simulink model "fuerza"  (R2020a)
settings: Solver=VariableStepAuto  StartTime=0.0  StopTime=2.5  RelTol=1e-3
values from neighbouring files (symbols this model uses):
  fd = 10/sqrt(2)*[1 1]    [init_control_fuerza.m]
  Ke = 1000    [init_control_fuerza.m]
  Kpf = (2*pi*freq)^2    (= 3947.84176044)    [init_control_fuerza.m]
  Kvf = 2*sqrt(Kpf)    [init_control_fuerza.m]
  Robot = Robot.perturb(0.8)    [init_control_fuerza.m]
undefined symbols (not defined in the file or in its folder): coriolis
libraries: roblocks x15, simulink x1
settings Model: Creator=Gianfranco  LastModifiedBy=Facu Molina

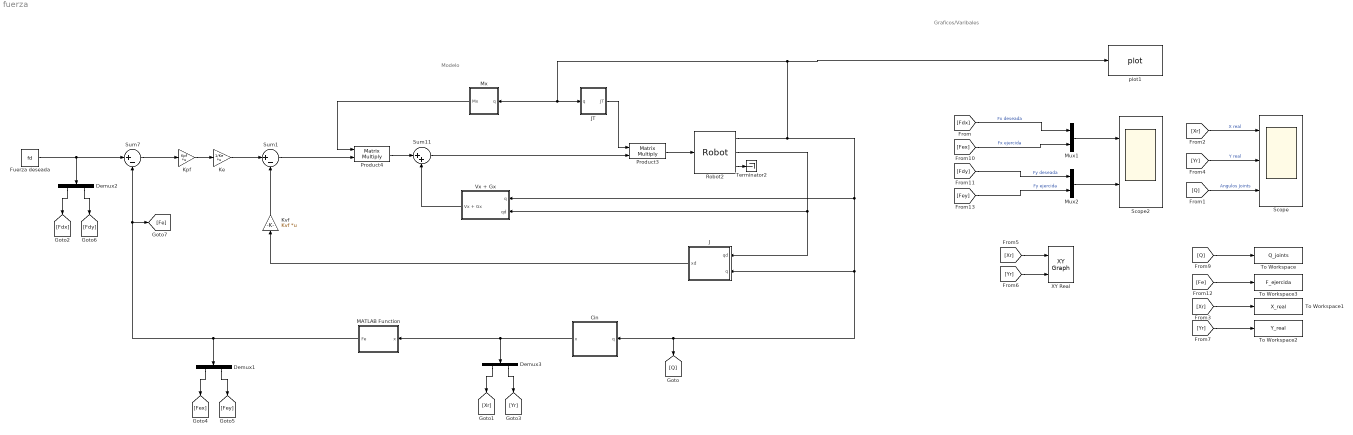
== system fuerza ==
  note: Graficos/Varibales
  note: Modelo
  Cin : Subsystem
  Demux1 : Demux  Outputs=2
  Demux2 : Demux  Outputs=2
  Demux3 : Demux  Outputs=2
  Fuerza deseada : Constant  Value=fd
  J : Subsystem
  JT : Subsystem
  Ke : Gain  Gain=1/Ke  Multiplication=Matrix(K*u)  SaturateOnIntegerOverflow=on  OutDataTypeStr=Inherit: Same as input  ParamDataTypeStr=Inherit: Same as input
  Kpf : Gain  Gain=Kpf  Multiplication=Matrix(K*u)  SaturateOnIntegerOverflow=on  OutDataTypeStr=Inherit: Same as input  ParamDataTypeStr=Inherit: Same as input
  Kvf : Gain  Gain=Kvf  Multiplication=Matrix(K*u)  SaturateOnIntegerOverflow=on  OutDataTypeStr=Inherit: Same as input  ParamDataTypeStr=Inherit: Same as input
  MATLAB Function : MATLAB Function  TreatAsAtomicUnit=on
  Mux1 : Mux  Inputs=2
  Mux2 : Mux  Inputs=2
  Mx : Subsystem
  Product3 : Product  Multiplication=Matrix(*)
  Product4 : Product  Multiplication=Matrix(*)
  Robot2 : roblocks/Arm/Robot  robot=Robot  q0=q0
      link override Integrator: InitialCondition=0
  Scope : Scope  NumInputPorts=3
  Scope2 : Scope  NumInputPorts=2
  Sum1 : Sum  Inputs=|+-  InputSameDT=on  SaturateOnIntegerOverflow=on  OutDataTypeStr=Inherit: Same as first input
  Sum11 : Sum  Inputs=|++  InputSameDT=on  SaturateOnIntegerOverflow=on  OutDataTypeStr=Inherit: Same as first input
  Sum7 : Sum  Inputs=|+-  InputSameDT=on  SaturateOnIntegerOverflow=on  OutDataTypeStr=Inherit: Same as first input
  Terminator2 : Terminator
  To Workspace : ToWorkspace  VariableName=Q_joints  SaveFormat=Timeseries  SampleTime=-1
  To Workspace1 : ToWorkspace  VariableName=X_real  SaveFormat=Timeseries  SampleTime=-1
  To Workspace2 : ToWorkspace  VariableName=Y_real  SaveFormat=Timeseries  SampleTime=-1
  To Workspace3 : ToWorkspace  VariableName=F_ejercida  SaveFormat=Timeseries  SampleTime=-1
  Vx + Gx : Subsystem
  XY Real : simulink/Sinks/XY Graph  xmin=-2  xmax=2  ymin=-2  ymax=2  st=-1
  plot1 : roblocks/Arm/plot  robot=Robot  fps=30  holdplot=on
  wires:
  Product3/1 -> Robot2/1
  Sum7/1 -> Kpf/1
  Product4/1 -> Sum11/1
  Robot2/3 -> Terminator2/1
  Mx/1(Mx) -> Product4/1
  Sum11/1 -> Product3/2
  JT/1(JT) -> Product3/1
  Robot2/2 -> Vx + Gx/2(qd), J/1(qd)
  Robot2/1 -> [Q], Cin/1(q), J/2(q), Vx + Gx/1(q), JT/1(q), Mx/1(q), plot1/1
  Vx + Gx/1(Vx + Gx) -> Sum11/2
  J/1(xd) -> Kvf/1
  [Xr] -> Scope/1  "X real"
  [Yr] -> Scope/2  "Y real"
  [Q] -> Scope/3  "Angulos Joints"
  [Xr] -> XY Real/1
  [Yr] -> XY Real/2
  [Q] -> To Workspace/1
  [Fe] -> To Workspace3/1
  Kpf/1 -> Ke/1
  Sum1/1 -> Product4/2
  Demux3/2 -> [Yr]
  Demux3/1 -> [Xr]
  Cin/1(x) -> MATLAB Function/1(x), Demux3/1
  [Fey] -> Mux2/2  "Fy ejercida"
  [Fdx] -> Mux1/1  "Fx deseada"
  [Fdy] -> Mux2/1  "Fy deseada"
  [Fex] -> Mux1/2  "Fx ejercida"
  Mux2/1 -> Scope2/2
  Mux1/1 -> Scope2/1
  Demux1/2 -> [Fey]
  Demux1/1 -> [Fex]
  Demux2/1 -> [Fdx]
  Demux2/2 -> [Fdy]
  Fuerza deseada/1 -> Demux2/1, Sum7/1
  MATLAB Function/1(Fe) -> Demux1/1, [Fe], Sum7/2
  Kvf/1 -> Sum1/2
  Ke/1 -> Sum1/1
  [Xr] -> To Workspace1/1
  [Yr] -> To Workspace2/1

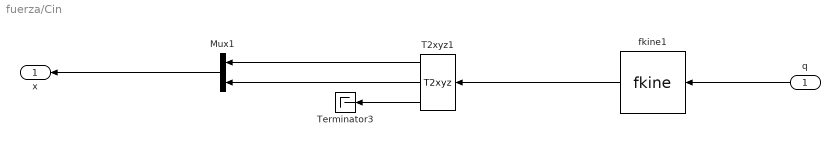
== system fuerza/Cin ==
  q : Inport
  Mux1 : Mux  Inputs=2
  T2xyz1 : roblocks/Toolbox/T2xyz
  Terminator3 : Terminator
  fkine1 : roblocks/Arm/fkine  robot=Robot
  x : Outport
  wires:
  T2xyz1/3 -> Terminator3/1
  fkine1/1 -> T2xyz1/1
  Mux1/1 -> x/1
  T2xyz1/2 -> Mux1/2
  T2xyz1/1 -> Mux1/1
  q/1 -> fkine1/1

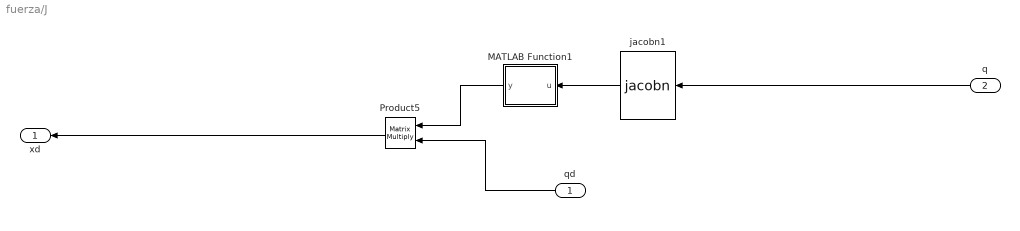
== system fuerza/J ==
  qd : Inport
  q : Inport  Port=2
  MATLAB Function1 : MATLAB Function  TreatAsAtomicUnit=on
  Product5 : Product  Multiplication=Matrix(*)
  jacobn1 : roblocks/Arm/jacobn  robot=Robot
  xd : Outport
  wires:
  jacobn1/1 -> MATLAB Function1/1(u)
  Product5/1 -> xd/1
  MATLAB Function1/1(y) -> Product5/1
  qd/1 -> Product5/2
  q/1 -> jacobn1/1

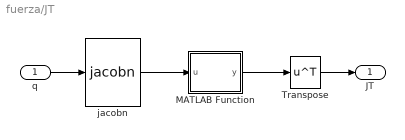
== system fuerza/JT ==
  q : Inport
  MATLAB Function : MATLAB Function  TreatAsAtomicUnit=on
  Transpose : Math  Operator=transpose  SaturateOnIntegerOverflow=on
  jacobn : roblocks/Arm/jacobn  robot=Robot
  JT : Outport
  wires:
  q/1 -> jacobn/1
  jacobn/1 -> MATLAB Function/1(u)
  Transpose/1 -> JT/1
  MATLAB Function/1(y) -> Transpose/1

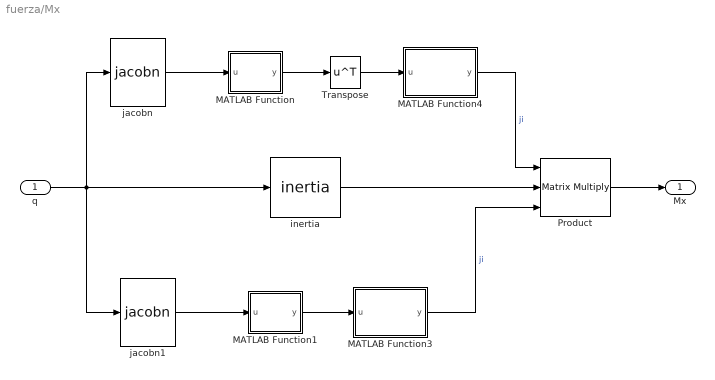
== system fuerza/Mx ==
  q : Inport
  MATLAB Function : MATLAB Function  TreatAsAtomicUnit=on
  MATLAB Function1 : MATLAB Function  TreatAsAtomicUnit=on
  MATLAB Function3 : MATLAB Function  TreatAsAtomicUnit=on
  MATLAB Function4 : MATLAB Function  TreatAsAtomicUnit=on
  Product : Product  Inputs=3  Multiplication=Matrix(*)
  Transpose : Math  Operator=transpose  SaturateOnIntegerOverflow=on
  inertia : roblocks/Arm/inertia  robot=Robot
  jacobn : roblocks/Arm/jacobn  robot=Robot
  jacobn1 : roblocks/Arm/jacobn  robot=Robot
  Mx : Outport
  wires:
  q/1 -> jacobn1/1, inertia/1, jacobn/1
  jacobn1/1 -> MATLAB Function1/1(u)
  Product/1 -> Mx/1
  inertia/1 -> Product/2
  jacobn/1 -> MATLAB Function/1(u)
  Transpose/1 -> MATLAB Function4/1(u)
  MATLAB Function/1(y) -> Transpose/1
  MATLAB Function3/1(y) -> Product/3  "ji"
  MATLAB Function1/1(y) -> MATLAB Function3/1(u)
  MATLAB Function4/1(y) -> Product/1  "ji"

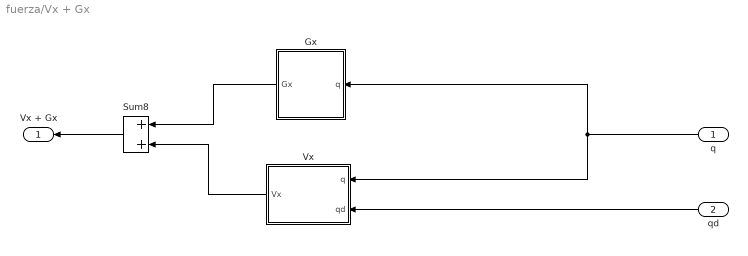
== system fuerza/Vx + Gx ==
  q : Inport
  qd : Inport  Port=2
  Gx : Subsystem
  Sum8 : Sum
  Vx : Subsystem
  Vx + Gx : Outport
  wires:
  Gx/1(Gx) -> Sum8/1
  Vx/1(Vx) -> Sum8/2
  Sum8/1 -> Vx + Gx/1
  qd/1 -> Vx/2(qd)
  q/1 -> Gx/1(q), Vx/1(q)

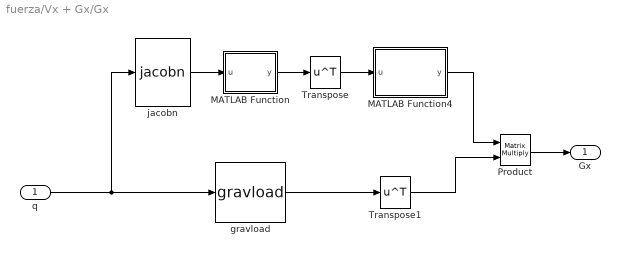
== system fuerza/Vx + Gx/Gx ==
  q : Inport
  MATLAB Function : MATLAB Function  TreatAsAtomicUnit=on
  MATLAB Function4 : MATLAB Function  TreatAsAtomicUnit=on
  Product : Product  Multiplication=Matrix(*)
  Transpose : Math  Operator=transpose  SaturateOnIntegerOverflow=on
  Transpose1 : Math  Operator=transpose  SaturateOnIntegerOverflow=on
  gravload : roblocks/Arm/gravload  robot=Robot
  jacobn : roblocks/Arm/jacobn  robot=Robot
  Gx : Outport
  wires:
  q/1 -> gravload/1, jacobn/1
  Product/1 -> Gx/1
  gravload/1 -> Transpose1/1
  jacobn/1 -> MATLAB Function/1(u)
  Transpose1/1 -> Product/2
  MATLAB Function/1(y) -> Transpose/1
  Transpose/1 -> MATLAB Function4/1(u)
  MATLAB Function4/1(y) -> Product/1

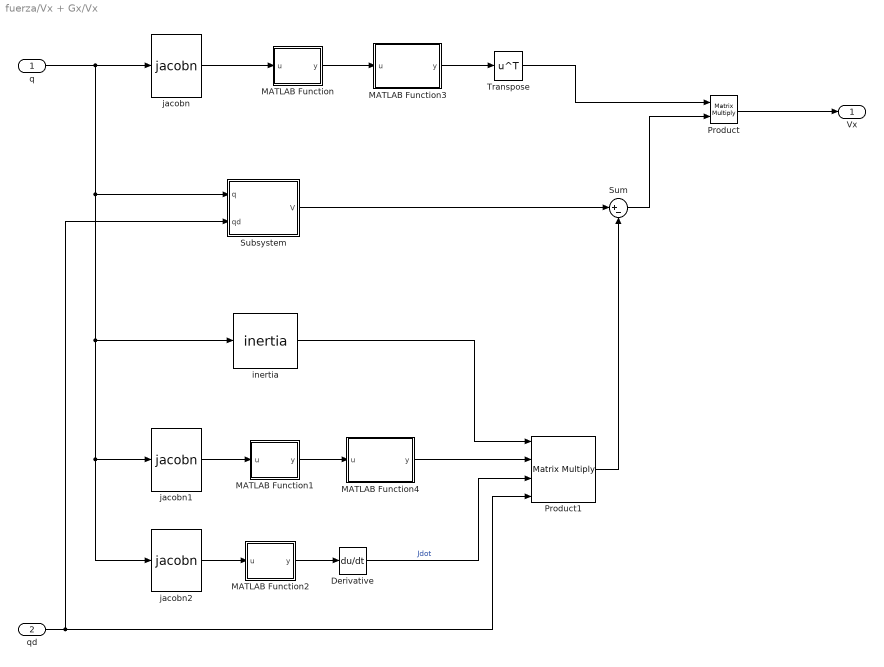
== system fuerza/Vx + Gx/Vx ==
  q : Inport
  qd : Inport  Port=2
  Derivative : Derivative
  MATLAB Function : MATLAB Function  TreatAsAtomicUnit=on
  MATLAB Function1 : MATLAB Function  TreatAsAtomicUnit=on
  MATLAB Function2 : MATLAB Function  TreatAsAtomicUnit=on
  MATLAB Function3 : MATLAB Function  TreatAsAtomicUnit=on
  MATLAB Function4 : MATLAB Function  TreatAsAtomicUnit=on
  Product : Product  Multiplication=Matrix(*)
  Product1 : Product  Inputs=4  Multiplication=Matrix(*)
  Subsystem : Subsystem
  Sum : Sum  Inputs=|+-
  Transpose : Math  Operator=transpose  SaturateOnIntegerOverflow=on
  inertia : roblocks/Arm/inertia  robot=Robot
  jacobn : roblocks/Arm/jacobn  robot=Robot
  jacobn1 : roblocks/Arm/jacobn  robot=Robot
  jacobn2 : roblocks/Arm/jacobn  robot=Robot
  Vx : Outport
  wires:
  MATLAB Function3/1(y) -> Transpose/1
  MATLAB Function/1(y) -> MATLAB Function3/1(u)
  jacobn/1 -> MATLAB Function/1(u)
  Sum/1 -> Product/2
  jacobn1/1 -> MATLAB Function1/1(u)
  MATLAB Function1/1(y) -> MATLAB Function4/1(u)
  jacobn2/1 -> MATLAB Function2/1(u)
  MATLAB Function2/1(y) -> Derivative/1
  inertia/1 -> Product1/1
  MATLAB Function4/1(y) -> Product1/2
  Derivative/1 -> Product1/3  "Jdot"
  Product1/1 -> Sum/2
  Transpose/1 -> Product/1
  Product/1 -> Vx/1
  Subsystem/1(V) -> Sum/1
  q/1 -> Subsystem/1(q), inertia/1, jacobn2/1, jacobn1/1, jacobn/1
  qd/1 -> Subsystem/2(qd), Product1/4

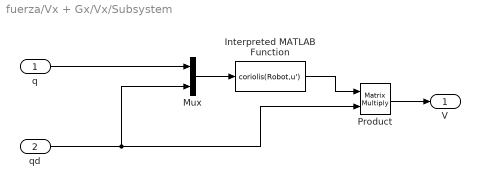
== system fuerza/Vx + Gx/Vx/Subsystem ==
  q : Inport
  qd : Inport  Port=2
  Interpreted MATLAB Function : MATLABFcn  MATLABFcn=coriolis(Robot,u')  OutputDimensions=[2,2]  Output1D=off
  Mux : Mux  Inputs=2
  Product : Product  Multiplication=Matrix(*)
  V : Outport
  wires:
  Product/1 -> V/1
  Interpreted MATLAB Function/1 -> Product/1
  Mux/1 -> Interpreted MATLAB Function/1
  q/1 -> Mux/1
  qd/1 -> Mux/2, Product/2

== matlab function fuerza/MATLAB Function ==
  data: x input; Fe output
function Fe = ModeloFuerza(x)
a = -1; %pendiente
b = 2; %ordenada al origen
ke = 1000;

y_limit =x(1)*a+b;
x_limit = (x(2)-b)/a;

if((x(1)<x_limit)&&(x(2)<y_limit))
    Fe=[0 0]';
else
    dist = abs(a*x(1)+2-x(2))/sqrt(a^2+1);
    Fe = [dist*ke/sqrt(2) dist*ke/sqrt(2)]';
end

== matlab function fuerza/Mx/MATLAB Function4 ==
  data: u input; y output
function y = pseudoinv(u)

y = pinv(u);

== matlab function fuerza/Vx + Gx/Gx/MATLAB Function4 ==
  data: u input; y output
function y = pseudoinv(u)

y = pinv(u);

== matlab function fuerza/Vx + Gx/Vx/MATLAB Function4 ==
  data: u input; y output
function y = pseudoinv(u)

y = pinv(u);

== matlab function fuerza/Vx + Gx/Vx/MATLAB Function3 ==
  data: u input; y output
function y = pseudoinv(u)

y = pinv(u);

== matlab function fuerza/JT/MATLAB Function ==
  data: u input; y output
function y = reshape(u)

y = u(1:2,1:2);

== matlab function fuerza/Mx/MATLAB Function ==
  data: u input; y output
function y = reshape(u)

y = u(1:2,1:2);

== matlab function fuerza/Mx/MATLAB Function3 ==
  data: u input; y output
function y = pseudoinv(u)

y = pinv(u);

== matlab function fuerza/Mx/MATLAB Function1 ==
  data: u input; y output
function y = reshape(u)

y = u(1:2,1:2);

== matlab function fuerza/Vx + Gx/Gx/MATLAB Function ==
  data: u input; y output
function y = reshape(u)

y = u(1:2,1:2);

== matlab function fuerza/J/MATLAB Function1 ==
  data: u input; y output
function y = reshape(u)

y = u(1:2,1:2);

== matlab function fuerza/Vx + Gx/Vx/MATLAB Function ==
  data: u input; y output
function y = reshape(u)

y = u(1:2,1:2);

== matlab function fuerza/Vx + Gx/Vx/MATLAB Function1 ==
  data: u input; y output
function y = reshape(u)

y = u(1:2,1:2);

== matlab function fuerza/Vx + Gx/Vx/MATLAB Function2 ==
  data: u input; y output
function y = reshape(u)

y = u(1:2,1:2);
